simulink model "Kalman_model"  (R2013a)
settings: Solver=ode45  StartTime=0.0  StopTime=10.0  RelTol=1e-3
values from neighbouring files (symbols this model uses):
  gamma = diag([1 1])    [Kalman_Filter.m]
  K = sigma * A*P*inv(s)    [Brid_code.m]    (also in Kalman_Filter.m = A_d*P*inv(s))
undefined symbols (not defined in the file or in its folder): A_d, B_d, C_d, e, v
settings Model: Creator=user  LastModifiedBy=user

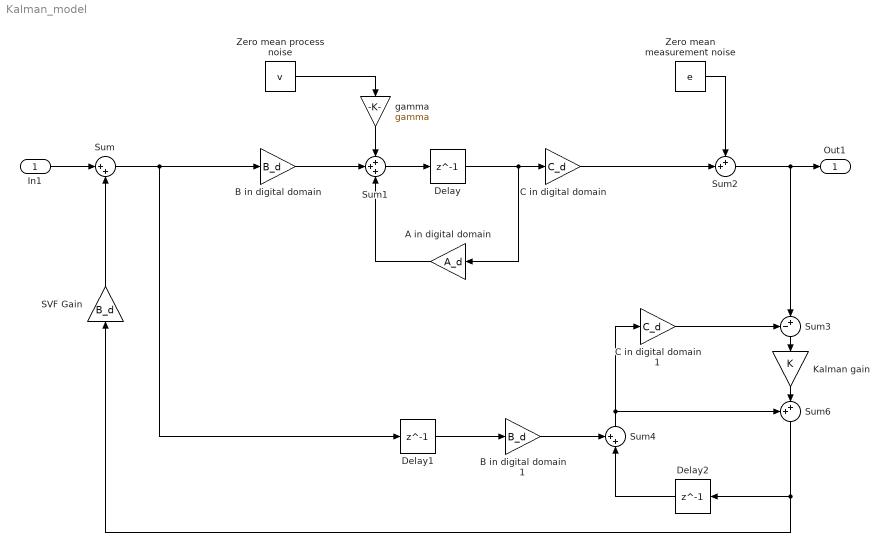
== system Kalman_model ==
  In1 : Inport
  A in digital domain : Gain  Gain=A_d
  "B in digital domain " : Gain  Gain=B_d
  B in digital domain 1 : Gain  Gain=B_d
  "C in digital domain " : Gain  Gain=C_d
  C in digital domain 1 : Gain  Gain=C_d
  Delay : Delay  DelayLength=1  InitialCondition=0
  Delay1 : Delay  DelayLength=1  InitialCondition=0
  Delay2 : Delay  DelayLength=1  InitialCondition=0
  Kalman gain : Gain  Gain=K
  SVF Gain : Gain  Gain=B_d
  Sum : Sum  Inputs=|++
  Sum1 : Sum  Inputs=+++
  Sum2 : Sum  Inputs=++|
  Sum3 : Sum  Inputs=-+|
  Sum4 : Sum  Inputs=++|
  Sum6 : Sum  Inputs=++|
  Zero mean measurement noise : Constant  Value=e
  Zero mean process noise : Constant  Value=v
  gamma : Gain  Gain=gamma
  Out1 : Outport
  wires:
  "B in digital domain "/1 -> Sum1/2
  A in digital domain/1 -> Sum1/3
  Sum1/1 -> Delay/1
  gamma/1 -> Sum1/1
  Delay/1 -> A in digital domain/1, "C in digital domain "/1
  In1/1 -> Sum/1
  "C in digital domain "/1 -> Sum2/2
  Sum2/1 -> Sum3/2, Out1/1
  Zero mean measurement noise/1 -> Sum2/1
  Zero mean process noise/1 -> gamma/1
  C in digital domain 1/1 -> Sum3/1
  Sum3/1 -> Kalman gain/1
  Delay1/1 -> B in digital domain 1/1
  Sum/1 -> Delay1/1, "B in digital domain "/1
  B in digital domain 1/1 -> Sum4/1
  Sum4/1 -> C in digital domain 1/1, Sum6/1
  Kalman gain/1 -> Sum6/2
  Delay2/1 -> Sum4/2
  SVF Gain/1 -> Sum/2
  Sum6/1 -> SVF Gain/1, Delay2/1
